simulink model "simulation_ex_5_2014a"  (R2014a)
settings: Solver=ode45  SolverMode=SingleTasking  StartTime=0.0  StopTime=10000  RelTol=1e-3
settings Model: CovMetricSettings=dwe  CovHtmlReporting=off  covSaveCumulativeToWorkspaceVar=off  CovSaveSingleToWorkspaceVar=off  CovExternalEMLEnable=on  CovSFcnEnable=on  Creator=HanO  LastModifiedBy=HanO
settings DataIOCC: LimitDataPoints=off  SaveFormat=StructureWithTime  ReturnWorkspaceOutputs=on
settings DebuggingCC: MergeDetectMultiDrivingBlocksExec=error  SolverPrmCheckMsg=none  FrameProcessingCompatibilityMsg=error  SFUnexpectedBacktrackingDiag=error  SFNoUnconditionalDefaultTransitionDiag=error
settings HardwareCC: ProdBitPerPointer=64  ProdLargestAtomicFloat=Float  ProdIntDivRoundTo=Zero  ProdEndianess=LittleEndian  ProdHWDeviceType=Specified
settings ModelReferenceCC: PropagateSignalLabelsOutOfModel=on
settings SFSimCC: SimUseLocalCustomCode=on
settings RTWCC: RTWUseLocalCustomCode=on
settings GRTTargetCC: TargetLangStandard=C99 (ISO)

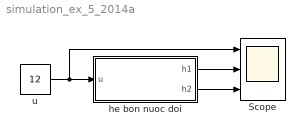
== system simulation_ex_5_2014a ==
  Scope : Scope  NumInputPorts=3
      settings: TimeRange=auto  MaxDataPoints=5000  SaveName=ScopeData  YMin=2.00000~-5.73394~-15.92762  YMax=22.00000~51.6055~143.3486  SampleTime=-1
  he bon nuoc doi : Subsystem  mask{AA1=10, AA2=15, k=0.5, a1=0.5, a2=0.2, cd1=0.4, cd2=0.6, g=9.81, h1_zero=0, h2_zero=0}
      mask prompts: AA1 "Tiết diện ngang bồn 1"; AA2 "Tiết diện ngang bồn 2"; k "Hệ số công suất máy bơm"; a1 "Tiết diện valve xả bồn 1"; a2 "Tiết diện valve xả bồn 2"; cd1 "Hệ số xả valve bồn 1"; cd2 "Hệ số xả valve bồn 2"; g "Gia tốc trọng trường"; h1_zero "Chiều cao mực nước bồn 1 ban đầu"; h2_zero "Chiều cao mực nước bồn 2 ban đầu"
  u : Constant  Value=12
  wires:
  u/1 -> Scope/1, he bon nuoc doi/1(u)
  he bon nuoc doi/1(h1) -> Scope/2
  he bon nuoc doi/2(h2) -> Scope/3

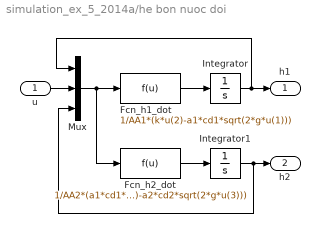
== system simulation_ex_5_2014a/he bon nuoc doi ==
  u : Inport
  Fcn_h1_dot : Fcn  Expr=1/AA1*(k*u(2)-a1*cd1*sqrt(2*g*u(1)))
  Fcn_h2_dot : Fcn  Expr=1/AA2*(a1*cd1*sqrt(2*g*u(1))-a2*cd2*sqrt(2*g*u(3)))
  Integrator : Integrator  InitialCondition=h1_zero
  Integrator1 : Integrator  InitialCondition=h2_zero
  Mux : Mux  Inputs=3
  h1 : Outport
  h2 : Outport  Port=2
  wires:
  Fcn_h1_dot/1 -> Integrator/1
  Fcn_h2_dot/1 -> Integrator1/1
  u/1 -> Mux/2
  Mux/1 -> Fcn_h2_dot/1, Fcn_h1_dot/1
  Integrator/1 -> Mux/1, h1/1
  Integrator1/1 -> h2/1, Mux/3
